simulink model "hexacopter_sim"  (R2023a)
settings: Solver=VariableStepAuto  StartTime=0.0  StopTime=15  MaxStep=0.001  RelTol=1e-7  EnableMultiTasking=on
values from neighbouring files (symbols this model uses):
  arm_length = 0.35    [hexacopter.m]    (also in hexacopter_unmodified.m)
  batteryDistanceFromCOG = -0.1    [hexacopter.m]    (also in hexacopter_unmodified.m)
  batteryMass = 0.56*2    (= 1.12)    [hexacopter.m]    (also in hexacopter_unmodified.m)
  batVolt = 3.7*cells    (= 14.8)    [hexacopter.m]    (also in hexacopter_unmodified.m)
  bodyMass = 1.2    [hexacopter.m]    (also in hexacopter_unmodified.m)
  deadCurrent = 0.3    [hexacopter.m]    (also in hexacopter_unmodified.m)
  droneMass = bodyMass + motorCount*(motorMass + propellerMassRaw)    (= 2.424)    [hexacopter.m]    (also in hexacopter_unmodified.m)
  h1al = 0.07    [discrete_controller_tuning.m]    (also in height_controller.m; hexacopter.m; hexacopter_unmodified.m)
  h1kp = 60    [hexacopter.m]    (also in hexacopter_unmodified.m)
  h1td = 1 / (sqrt(h1al) * target)    [height_controller.m]    (also in hexacopter.m = 1; hexacopter_unmodified.m = 1)
  h1ti = h1Ni * (1/ target)    (= 1.27118644068)    [height_controller.m]    (also in hexacopter.m = 1; hexacopter_unmodified.m = 1)
  h1val = 0.6    [discrete_controller_tuning.m]    (also in hexacopter.m = 0)
  h1vkp = 1    [hexacopter.m]
  h1vtd = 0    [hexacopter.m]
  h1vti = 1    [hexacopter.m]
  h_beta = 5    [hexacopter.m]    (also in hexacopter_unmodified.m)
  h_tau = 1.5    [hexacopter.m]    (also in hexacopter_unmodified.m)
  hoverControl = hoverVoltage/batVolt*1024    [hexacopter.m]    (also in hexacopter_unmodified.m)
  hoverVoltage = hoverCurrent * Ra + hoverRPM / Kv    [hexacopter.m]    (also in hexacopter_unmodified.m)
  KDrag = 1.5e-9    (= 1.5e-09)    [hexacopter.m]    (also in hexacopter_unmodified.m)
  Km = 60/(Kv * 2 * pi)    (= 0.013641852265)    [hexacopter.m]    (also in hexacopter_unmodified.m)
  Ktrust = 2.7e-5    (= 2.7e-05)    [hexacopter.m]    (also in hexacopter_unmodified.m)
  minimumMotorVolt = 1.0    (= 1)    [hexacopter.m]    (also in hexacopter_unmodified.m)
  motorMass = motorOnlyMass + 0.085    (= 0.187)    [hexacopter.m]    (also in hexacopter_unmodified.m)
  N = solve(eqn,V)    [temp.m]
  paal = 0.2    [hexacopter.m]    (also in hexacopter_unmodified.m)
  pakp = 0    [hexacopter.m]    (also in hexacopter_unmodified.m)
  pal = 0.5    [hexacopter.m]    (also in hexacopter_unmodified.m)
  patd = 1    [hexacopter.m]    (also in hexacopter_unmodified.m)
  pati = 100    [hexacopter.m]    (also in hexacopter_unmodified.m)
  pkp = 0    [hexacopter.m]    (also in hexacopter_unmodified.m)
  propellerMass = propellerMassRaw + 3*motorInertia/propellerRadius^2    (= 0.0220980494455)    [hexacopter.m]    (also in hexacopter_unmodified.m)
  ptd = 1    [hexacopter.m]    (also in hexacopter_unmodified.m)
  pti = 1    [hexacopter.m]    (also in hexacopter_unmodified.m)
  pushEnabled = 0    [hexacopter.m]    (also in hexacopter_unmodified.m)
  Ra = 0.083    [hexacopter.m]    (also in hexacopter_unmodified.m)
  raal = 0.2    [hexacopter.m]    (also in hexacopter_unmodified.m)
  rakp = 0    [hexacopter.m]    (also in hexacopter_unmodified.m)
  ral = 0.5    [hexacopter.m]    (also in hexacopter_unmodified.m)
  ratd = 1    [hexacopter.m]    (also in hexacopter_unmodified.m)
  rati = 100    [hexacopter.m]    (also in hexacopter_unmodified.m)
  rkp = 0    [hexacopter.m]    (also in hexacopter_unmodified.m)
  roll_limit = 10    [hexacopter.m]    (also in hexacopter_unmodified.m)
  rtd = 1    [hexacopter.m]    (also in hexacopter_unmodified.m)
  rti = 1    [hexacopter.m]    (also in hexacopter_unmodified.m)
  xal = 0.2    [hexacopter.m]    (also in hexacopter_unmodified.m = 1)
  xkp = 0    [hexacopter.m]    (also in hexacopter_unmodified.m)
  xtd = 1    [hexacopter.m]    (also in hexacopter_unmodified.m)
  xti = 100    [hexacopter.m]    (also in hexacopter_unmodified.m)
  xval = 0.2    [hexacopter.m]    (also in hexacopter_unmodified.m = 0.3; vel_controller.m = 0.3)
  xvkp = 0    [hexacopter.m]    (also in hexacopter_unmodified.m; vel_controller.m = 0.184077200147)
  xvtd = 1    [hexacopter.m]    (also in hexacopter_unmodified.m; vel_controller.m = 1 / (sqrt(xval) * target))
  xvti = 100    [hexacopter.m]    (also in hexacopter_unmodified.m; vel_controller.m = 0)
  yaal = 0.5    [hexacopter.m]    (also in hexacopter_unmodified.m)
  yakp = 0    [hexacopter.m]    (also in hexacopter_unmodified.m)
  yal = 0.5    [hexacopter.m]    (also in hexacopter_unmodified.m)
  yatd = 1    [hexacopter.m]    (also in hexacopter_unmodified.m)
  yati = 100    [hexacopter.m]    (also in hexacopter_unmodified.m)
  yaw_limit = 45    [hexacopter.m]    (also in hexacopter_unmodified.m)
  yiLim = 500    [hexacopter.m]    (also in hexacopter_unmodified.m)
  ykp = 0    [hexacopter.m]    (also in hexacopter_unmodified.m)
  ytd = 0    [hexacopter.m]    (also in hexacopter_unmodified.m)
  yti = 1000    [hexacopter.m]    (also in hexacopter_unmodified.m)
  yval = 0.3    [hexacopter.m]    (also in hexacopter_unmodified.m)
  yvkp = 0    [hexacopter.m]    (also in hexacopter_unmodified.m)
  yvtd = 1    [hexacopter.m]    (also in hexacopter_unmodified.m)
  yvti = 100    [hexacopter.m]    (also in hexacopter_unmodified.m)
undefined symbols (not defined in the file or in its folder): h2al, h2kp, h2td, h2ti, X, Y, Z
libraries: sm_lib x52, nesl_utility x34, simulink x3
(part 3 of 3)

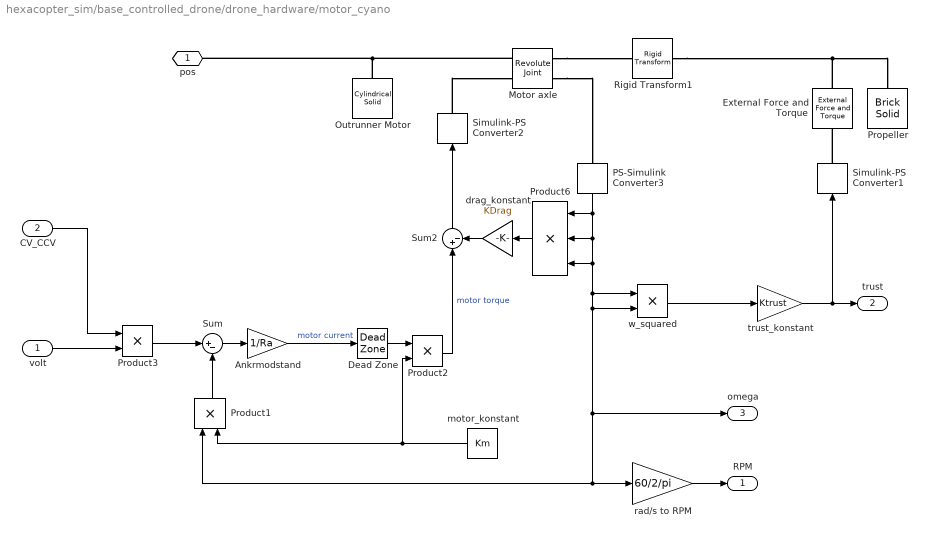
== system hexacopter_sim/base_controlled_drone/drone_hardware/motor_cyano ==
  volt : Inport
  CV_CCV : Inport  Port=2
  Ankrmodstand : Gain  Gain=1/Ra
  Dead Zone : DeadZone  LowerValue=-deadCurrent  UpperValue=deadCurrent
  External Force and Torque : sm_lib/Forces and Torques/External Force and Torque  ForceResolutionFrame=AttachedFrame  EnableForceX=off  EnableForceY=off  EnableForceZ=on  EnableForce=off  TorqueResolutionFrame=AttachedFrame  EnableTorqueX=off  EnableTorqueY=off  EnableTorqueZ=off  EnableTorque=off
  Motor axle : sm_lib/Joints/Revolute Joint  JointMode=Normal  SenseConstraintForce=off  SenseConstraintForceX=off  SenseConstraintForceY=off  SenseConstraintForceZ=off  SenseConstraintTorque=off  SenseConstraintTorqueX=off  SenseConstraintTorqueY=off  SenseConstraintTorqueZ=off  SenseTotalForce=off  SenseTotalForceX=off  SenseTotalForceY=off  SenseTotalForceZ=off  SenseTotalTorque=off  SenseTotalTorqueX=off  SenseTotalTorqueY=off  SenseTotalTorqueZ=off  CompositeWrenchDir=FollowerOnBase  CompositeWrenchFrame=BaseFrame  EquilibriumPosition=0  EquilibriumPositionUnits=deg  SpringStiffness=0  SpringStiffnessUnits=N*m/deg  DampingCoefficient=0  DampingCoefficientUnits=N*m/(deg/s)  TorqueActuationMode=InputTorque  MotionActuationMode=ComputedMotion  SensePosition=off  SenseVelocity=on  SenseAcceleration=off  SenseTorqueForce=off  SenseLowerLimitTorqueForce=off  SenseUpperLimitTorqueForce=off  LowerLimitSpecify=off  LowerLimitBound=-90  LowerLimitBoundUnits=deg  LowerLimitStiffness=1e4  LowerLimitStiffnessUnits=N*m/deg  LowerLimitDamping=10  LowerLimitDampingUnits=N*m/(deg/s)  LowerLimitTransitionRegionWidth=0.1  LowerLimitTransitionRegionWidthUnits=deg  UpperLimitSpecify=off  UpperLimitBound=90  UpperLimitBoundUnits=deg  UpperLimitStiffness=1e4  UpperLimitStiffnessUnits=N*m/deg  UpperLimitDamping=10  UpperLimitDampingUnits=N*m/(deg/s)  UpperLimitTransitionRegionWidth=0.1  UpperLimitTransitionRegionWidthUnits=deg  PositionTargetSpecify=off  PositionTargetPriority=High  PositionTargetValue=0  PositionTargetValueUnits=deg  VelocityTargetSpecify=on  VelocityTargetPriority=High  VelocityTargetValue=0  VelocityTargetValueUnits=rad/s
  Outrunner Motor : sm_lib/Body Elements/Cylindrical Solid  GraphicAmbientColor=[0.15 0.15 0.15 1.0]  BasedOnType=Mass  CenterOfMass=[0 0 0]  CenterOfMassUnits=m  GraphicDiffuseColor=[0.2 0.6 0.0]  CylinderLength=0.05  CylinderLengthUnits=m  CylinderRadius=0.02  CylinderRadiusUnits=m  Density=1000  DensityUnits=kg/(m^3)  DoExposeReferenceFrame=on  GraphicEmissiveColor=[0.0 0.0 0.0 1.0]  ExportEntireGeometry=off  SerializedFrames=<Frames/>  MarkerShape=Sphere  MarkerSize=10  GraphicType=FromGeometry  InertiaType=CalculateFromGeometry  Mass=motorMass  MassUnits=kg  MomentsOfInertia=[1 1 1]  MomentsOfInertiaUnits=kg*m^2  GraphicOpacity=1.0  ProductsOfInertia=[0 0 0]  ProductsOfInertiaUnits=kg*m^2  GraphicShininess=75  GraphicSpecularColor=[0.5 0.5 0.5 1.0]  GraphicVisPropType=SimpleVisualProperties
  PS-Simulink Converter3 : nesl_utility/PS-Simulink Converter  PhysicalDomain=network_engine_domain  SubClassName=ps_output  LeftPortType=input  RightPortType=output  PseudoPeriodic=off  Frequencies=[]  VectorFormat=1-D array  Unit=1  AffineConversion=off
  Product1 : Product
  Product2 : Product
  Product3 : Product
  Product6 : Product  Inputs=3
  Propeller : sm_lib/Body Elements/Brick Solid  GraphicAmbientColor=[0.15 0.15 0.15 1.0]  BasedOnType=Mass  BrickDimensions=[0.34 0.03 0.01]  BrickDimensionsUnits=m  CenterOfMass=[0 0 0]  CenterOfMassUnits=m  GraphicDiffuseColor=[0.0 0.8 0.8]  Density=1000  DensityUnits=kg/(m^3)  DoExposeReferenceFrame=on  GraphicEmissiveColor=[0.0 0.0 0.0 1.0]  ExportEntireGeometry=off  SerializedFrames=<Frames/>  MarkerShape=Sphere  MarkerSize=10  GraphicType=FromGeometry  InertiaType=CalculateFromGeometry  Mass=propellerMass  MassUnits=kg  MomentsOfInertia=[1 1 1]  MomentsOfInertiaUnits=kg*m^2  GraphicOpacity=1.0  ProductsOfInertia=[0 0 0]  ProductsOfInertiaUnits=kg*m^2  GraphicShininess=75  GraphicSpecularColor=[0.5 0.5 0.5 1.0]  GraphicVisPropType=SimpleVisualProperties
  Rigid Transform1 : sm_lib/Frames and Transforms/Rigid Transform  TranslationMethod=Cartesian  TranslationStandardOffset=0  TranslationStandardOffsetUnits=m  TranslationStandardAxis=+Z  TranslationCartesianOffset=[0 0 0.03]  TranslationCartesianOffsetUnits=m  TranslationROffset=0  TranslationROffsetUnits=m  TranslationZOffset=0  TranslationZOffsetUnits=m  TranslationThetaOffset=0  TranslationThetaOffsetUnits=deg  RotationMethod=StandardAxis  RotationAngleUnits=deg  RotationStandardAxis=+Z  RotationAngle=0.0  RotationArbitraryAxis=[0 0 1]  FollAlignAxisA=+X  BaseAlignAxisA=+Y  FollAlignAxisB=+Y  BaseAlignAxisB=+Z  RotationSequenceAxes=FollowerAxes  RotationSequence=XYX  RotationSequenceAngles=[0 0 0]  RotationSequenceAnglesUnits=deg  RotationMatrix=[1 0 0; 0 1 0; 0 0 1]  Quaternion=[1 0 0 0]
  Simulink-PS Converter1 : nesl_utility/Simulink-PS Converter  PhysicalDomain=network_engine_domain  SubClassName=ps_input  LeftPortType=input  RightPortType=output  PseudoPeriodic=off  Frequencies=[]  NoiseDistribution=none  NoiseParameters=[]  Unit=1  AffineConversion=off  FilteringAndDerivatives=zero  SimscapeFilterOrder=1  InputFilterTimeConstant=0.001  UdotUserProvided=1
  Simulink-PS Converter2 : nesl_utility/Simulink-PS Converter  PhysicalDomain=network_engine_domain  SubClassName=ps_input  LeftPortType=input  RightPortType=output  PseudoPeriodic=off  Frequencies=[]  NoiseDistribution=none  NoiseParameters=[]  Unit=1  AffineConversion=off  FilteringAndDerivatives=zero  SimscapeFilterOrder=1  InputFilterTimeConstant=0.001  UdotUserProvided=1
  Sum : Sum  Inputs=|+-
  Sum2 : Sum  Inputs=|+-
  drag_konstant : Gain  Gain=KDrag
  motor_konstant : Constant  Value=Km
  rad/s to RPM : Gain  Gain=60/2/pi
  trust_konstant : Gain  Gain=Ktrust
  w_squared : Product
  pos : PMIOPort  Side=Left
  RPM : Outport  VectorParamsAs1DForOutWhenUnconnected=off
  trust : Outport  Port=2  VectorParamsAs1DForOutWhenUnconnected=off
  omega : Outport  Port=3  VectorParamsAs1DForOutWhenUnconnected=off
  wires:
  rad/s to RPM/1 -> RPM/1
  motor_konstant/1 -> Product1/2, Product2/2
  Product1/1 -> Sum/2
  Product2/1 -> Sum2/1  "motor torque"
  Ankrmodstand/1 -> Dead Zone/1  "motor current"
  Sum/1 -> Ankrmodstand/1
  Sum2/1 -> Simulink-PS Converter2/1
  drag_konstant/1 -> Sum2/2
  volt/1 -> Product3/2
  Product3/1 -> Sum/1
  CV_CCV/1 -> Product3/1
  trust_konstant/1 -> trust/1, Simulink-PS Converter1/1
  w_squared/1 -> trust_konstant/1
  PS-Simulink Converter3/1 -> Product6/2, Product6/3, omega/1, rad/s to RPM/1, Product1/1, w_squared/2, w_squared/1, Product6/1
  Product6/1 -> drag_konstant/1
  Dead Zone/1 -> Product2/1
  connections:
  Simulink-PS Converter1/RConn1 -- External Force and Torque/LConn1
  Motor axle/RConn2 -- PS-Simulink Converter3/LConn1
  Motor axle/RConn1 -- Rigid Transform1/LConn1
  Simulink-PS Converter2/RConn1 -- Motor axle/LConn2
  Motor axle/LConn1 -- Outrunner Motor/RConn1 -- pos/RConn1
  External Force and Torque/RConn1 -- Propeller/RConn1 -- Rigid Transform1/RConn1

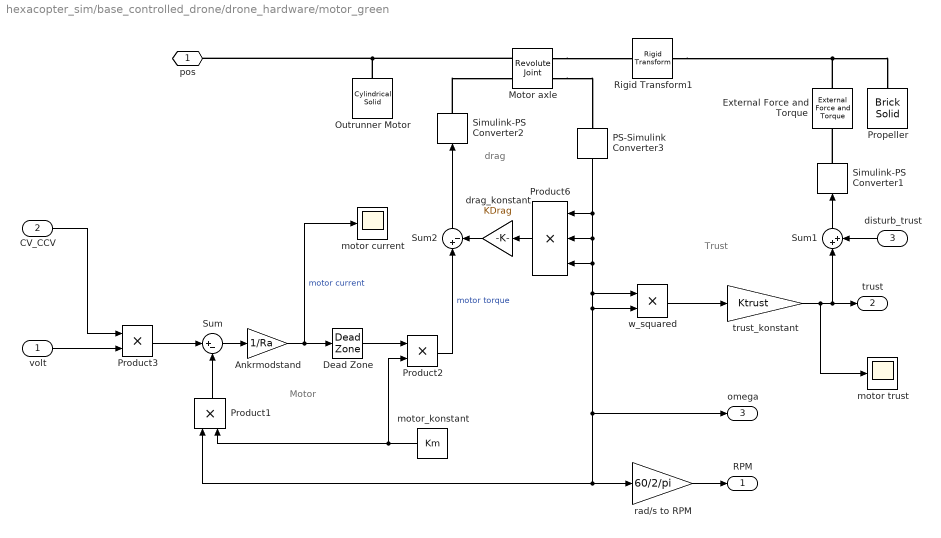
== system hexacopter_sim/base_controlled_drone/drone_hardware/motor_green ==
  note: drag
  note: Trust
  note: Motor
  volt : Inport
  CV_CCV : Inport  Port=2
  disturb_trust : Inport  Port=3
  Ankrmodstand : Gain  Gain=1/Ra
  Dead Zone : DeadZone  LowerValue=-deadCurrent  UpperValue=deadCurrent
  External Force and Torque : sm_lib/Forces and Torques/External Force and Torque  ForceResolutionFrame=AttachedFrame  EnableForceX=off  EnableForceY=off  EnableForceZ=on  EnableForce=off  TorqueResolutionFrame=AttachedFrame  EnableTorqueX=off  EnableTorqueY=off  EnableTorqueZ=off  EnableTorque=off
  Motor axle : sm_lib/Joints/Revolute Joint  JointMode=Normal  SenseConstraintForce=off  SenseConstraintForceX=off  SenseConstraintForceY=off  SenseConstraintForceZ=off  SenseConstraintTorque=off  SenseConstraintTorqueX=off  SenseConstraintTorqueY=off  SenseConstraintTorqueZ=off  SenseTotalForce=off  SenseTotalForceX=off  SenseTotalForceY=off  SenseTotalForceZ=off  SenseTotalTorque=off  SenseTotalTorqueX=off  SenseTotalTorqueY=off  SenseTotalTorqueZ=off  CompositeWrenchDir=FollowerOnBase  CompositeWrenchFrame=BaseFrame  EquilibriumPosition=0  EquilibriumPositionUnits=deg  SpringStiffness=0  SpringStiffnessUnits=N*m/deg  DampingCoefficient=0  DampingCoefficientUnits=N*m/(deg/s)  TorqueActuationMode=InputTorque  MotionActuationMode=ComputedMotion  SensePosition=off  SenseVelocity=on  SenseAcceleration=off  SenseTorqueForce=off  SenseLowerLimitTorqueForce=off  SenseUpperLimitTorqueForce=off  LowerLimitSpecify=off  LowerLimitBound=-90  LowerLimitBoundUnits=deg  LowerLimitStiffness=1e4  LowerLimitStiffnessUnits=N*m/deg  LowerLimitDamping=10  LowerLimitDampingUnits=N*m/(deg/s)  LowerLimitTransitionRegionWidth=0.1  LowerLimitTransitionRegionWidthUnits=deg  UpperLimitSpecify=off  UpperLimitBound=90  UpperLimitBoundUnits=deg  UpperLimitStiffness=1e4  UpperLimitStiffnessUnits=N*m/deg  UpperLimitDamping=10  UpperLimitDampingUnits=N*m/(deg/s)  UpperLimitTransitionRegionWidth=0.1  UpperLimitTransitionRegionWidthUnits=deg  PositionTargetSpecify=off  PositionTargetPriority=High  PositionTargetValue=0  PositionTargetValueUnits=deg  VelocityTargetSpecify=on  VelocityTargetPriority=High  VelocityTargetValue=0  VelocityTargetValueUnits=rad/s
  Outrunner Motor : sm_lib/Body Elements/Cylindrical Solid  GraphicAmbientColor=[0.15 0.15 0.15 1.0]  BasedOnType=Mass  CenterOfMass=[0 0 0]  CenterOfMassUnits=m  GraphicDiffuseColor=[0.2 0.6 0.0]  CylinderLength=0.05  CylinderLengthUnits=m  CylinderRadius=0.02  CylinderRadiusUnits=m  Density=1000  DensityUnits=kg/(m^3)  DoExposeReferenceFrame=on  GraphicEmissiveColor=[0.0 0.0 0.0 1.0]  ExportEntireGeometry=off  SerializedFrames=<Frames/>  MarkerShape=Sphere  MarkerSize=10  GraphicType=FromGeometry  InertiaType=CalculateFromGeometry  Mass=motorMass  MassUnits=kg  MomentsOfInertia=[1 1 1]  MomentsOfInertiaUnits=kg*m^2  GraphicOpacity=1.0  ProductsOfInertia=[0 0 0]  ProductsOfInertiaUnits=kg*m^2  GraphicShininess=75  GraphicSpecularColor=[0.5 0.5 0.5 1.0]  GraphicVisPropType=SimpleVisualProperties
  PS-Simulink Converter3 : nesl_utility/PS-Simulink Converter  PhysicalDomain=network_engine_domain  SubClassName=ps_output  LeftPortType=input  RightPortType=output  PseudoPeriodic=off  Frequencies=[]  VectorFormat=1-D array  Unit=1  AffineConversion=off
  Product1 : Product
  Product2 : Product
  Product3 : Product
  Product6 : Product  Inputs=3
  Propeller : sm_lib/Body Elements/Brick Solid  GraphicAmbientColor=[0.15 0.15 0.15 1.0]  BasedOnType=Mass  BrickDimensions=[0.34 0.03 0.01]  BrickDimensionsUnits=m  CenterOfMass=[0 0 0]  CenterOfMassUnits=m  GraphicDiffuseColor=[0.0 0.8 0.0]  Density=1000  DensityUnits=kg/(m^3)  DoExposeReferenceFrame=on  GraphicEmissiveColor=[0.0 0.0 0.0 1.0]  ExportEntireGeometry=off  SerializedFrames=<Frames/>  MarkerShape=Sphere  MarkerSize=10  GraphicType=FromGeometry  InertiaType=CalculateFromGeometry  Mass=propellerMass  MassUnits=kg  MomentsOfInertia=[1 1 1]  MomentsOfInertiaUnits=kg*m^2  GraphicOpacity=1.0  ProductsOfInertia=[0 0 0]  ProductsOfInertiaUnits=kg*m^2  GraphicShininess=75  GraphicSpecularColor=[0.5 0.5 0.5 1.0]  GraphicVisPropType=SimpleVisualProperties
  Rigid Transform1 : sm_lib/Frames and Transforms/Rigid Transform  TranslationMethod=Cartesian  TranslationStandardOffset=0  TranslationStandardOffsetUnits=m  TranslationStandardAxis=+Z  TranslationCartesianOffset=[0 0 0.03]  TranslationCartesianOffsetUnits=m  TranslationROffset=0  TranslationROffsetUnits=m  TranslationZOffset=0  TranslationZOffsetUnits=m  TranslationThetaOffset=0  TranslationThetaOffsetUnits=deg  RotationMethod=StandardAxis  RotationAngleUnits=deg  RotationStandardAxis=+Z  RotationAngle=0.0  RotationArbitraryAxis=[0 0 1]  FollAlignAxisA=+X  BaseAlignAxisA=+Y  FollAlignAxisB=+Y  BaseAlignAxisB=+Z  RotationSequenceAxes=FollowerAxes  RotationSequence=XYX  RotationSequenceAngles=[0 0 0]  RotationSequenceAnglesUnits=deg  RotationMatrix=[1 0 0; 0 1 0; 0 0 1]  Quaternion=[1 0 0 0]
  Simulink-PS Converter1 : nesl_utility/Simulink-PS Converter  PhysicalDomain=network_engine_domain  SubClassName=ps_input  LeftPortType=input  RightPortType=output  PseudoPeriodic=off  Frequencies=[]  NoiseDistribution=none  NoiseParameters=[]  Unit=1  AffineConversion=off  FilteringAndDerivatives=zero  SimscapeFilterOrder=1  InputFilterTimeConstant=0.001  UdotUserProvided=1
  Simulink-PS Converter2 : nesl_utility/Simulink-PS Converter  PhysicalDomain=network_engine_domain  SubClassName=ps_input  LeftPortType=input  RightPortType=output  PseudoPeriodic=off  Frequencies=[]  NoiseDistribution=none  NoiseParameters=[]  Unit=1  AffineConversion=off  FilteringAndDerivatives=zero  SimscapeFilterOrder=1  InputFilterTimeConstant=0.001  UdotUserProvided=1
  Sum : Sum  Inputs=|+-
  Sum1 : Sum  Inputs=|++
  Sum2 : Sum  Inputs=|+-
  drag_konstant : Gain  Gain=KDrag
  motor current : Scope
  motor trust : Scope
  motor_konstant : Constant  Value=Km
  rad/s to RPM : Gain  Gain=60/2/pi
  trust_konstant : Gain  Gain=Ktrust
  w_squared : Product
  pos : PMIOPort  Side=Left
  RPM : Outport  VectorParamsAs1DForOutWhenUnconnected=off
  trust : Outport  Port=2  VectorParamsAs1DForOutWhenUnconnected=off
  omega : Outport  Port=3  VectorParamsAs1DForOutWhenUnconnected=off
  wires:
  rad/s to RPM/1 -> RPM/1
  motor_konstant/1 -> Product1/2, Product2/2
  Product1/1 -> Sum/2
  trust_konstant/1 -> motor trust/1, Sum1/1, trust/1
  Product2/1 -> Sum2/1  "motor torque"
  Ankrmodstand/1 -> motor current/1, Dead Zone/1  "motor current"
  Sum/1 -> Ankrmodstand/1
  Sum2/1 -> Simulink-PS Converter2/1
  drag_konstant/1 -> Sum2/2
  volt/1 -> Product3/2
  Product3/1 -> Sum/1
  CV_CCV/1 -> Product3/1
  Sum1/1 -> Simulink-PS Converter1/1
  disturb_trust/1 -> Sum1/2
  w_squared/1 -> trust_konstant/1
  PS-Simulink Converter3/1 -> omega/1, rad/s to RPM/1, Product1/1, w_squared/2, w_squared/1, Product6/3, Product6/2, Product6/1
  Product6/1 -> drag_konstant/1
  Dead Zone/1 -> Product2/1
  connections:
  Simulink-PS Converter1/RConn1 -- External Force and Torque/LConn1
  Motor axle/RConn2 -- PS-Simulink Converter3/LConn1
  Motor axle/RConn1 -- Rigid Transform1/LConn1
  Simulink-PS Converter2/RConn1 -- Motor axle/LConn2
  Motor axle/LConn1 -- Outrunner Motor/RConn1 -- pos/RConn1
  External Force and Torque/RConn1 -- Propeller/RConn1 -- Rigid Transform1/RConn1

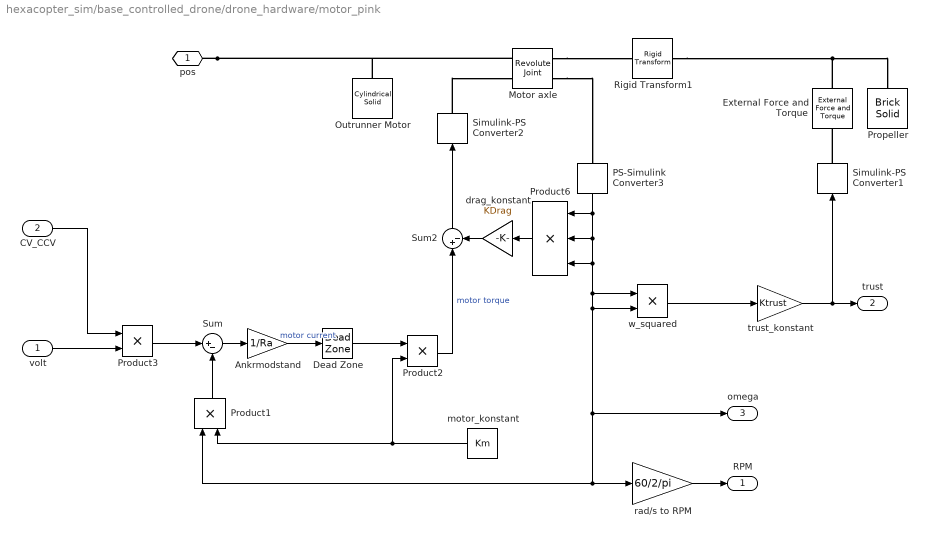
== system hexacopter_sim/base_controlled_drone/drone_hardware/motor_pink ==
  volt : Inport
  CV_CCV : Inport  Port=2
  Ankrmodstand : Gain  Gain=1/Ra
  Dead Zone : DeadZone  LowerValue=-deadCurrent  UpperValue=deadCurrent
  External Force and Torque : sm_lib/Forces and Torques/External Force and Torque  ForceResolutionFrame=AttachedFrame  EnableForceX=off  EnableForceY=off  EnableForceZ=on  EnableForce=off  TorqueResolutionFrame=AttachedFrame  EnableTorqueX=off  EnableTorqueY=off  EnableTorqueZ=off  EnableTorque=off
  Motor axle : sm_lib/Joints/Revolute Joint  JointMode=Normal  SenseConstraintForce=off  SenseConstraintForceX=off  SenseConstraintForceY=off  SenseConstraintForceZ=off  SenseConstraintTorque=off  SenseConstraintTorqueX=off  SenseConstraintTorqueY=off  SenseConstraintTorqueZ=off  SenseTotalForce=off  SenseTotalForceX=off  SenseTotalForceY=off  SenseTotalForceZ=off  SenseTotalTorque=off  SenseTotalTorqueX=off  SenseTotalTorqueY=off  SenseTotalTorqueZ=off  CompositeWrenchDir=FollowerOnBase  CompositeWrenchFrame=BaseFrame  EquilibriumPosition=0  EquilibriumPositionUnits=deg  SpringStiffness=0  SpringStiffnessUnits=N*m/deg  DampingCoefficient=0  DampingCoefficientUnits=N*m/(deg/s)  TorqueActuationMode=InputTorque  MotionActuationMode=ComputedMotion  SensePosition=off  SenseVelocity=on  SenseAcceleration=off  SenseTorqueForce=off  SenseLowerLimitTorqueForce=off  SenseUpperLimitTorqueForce=off  LowerLimitSpecify=off  LowerLimitBound=-90  LowerLimitBoundUnits=deg  LowerLimitStiffness=1e4  LowerLimitStiffnessUnits=N*m/deg  LowerLimitDamping=10  LowerLimitDampingUnits=N*m/(deg/s)  LowerLimitTransitionRegionWidth=0.1  LowerLimitTransitionRegionWidthUnits=deg  UpperLimitSpecify=off  UpperLimitBound=90  UpperLimitBoundUnits=deg  UpperLimitStiffness=1e4  UpperLimitStiffnessUnits=N*m/deg  UpperLimitDamping=10  UpperLimitDampingUnits=N*m/(deg/s)  UpperLimitTransitionRegionWidth=0.1  UpperLimitTransitionRegionWidthUnits=deg  PositionTargetSpecify=off  PositionTargetPriority=High  PositionTargetValue=0  PositionTargetValueUnits=deg  VelocityTargetSpecify=on  VelocityTargetPriority=High  VelocityTargetValue=0  VelocityTargetValueUnits=rad/s
  Outrunner Motor : sm_lib/Body Elements/Cylindrical Solid  GraphicAmbientColor=[0.15 0.15 0.15 1.0]  BasedOnType=Mass  CenterOfMass=[0 0 0]  CenterOfMassUnits=m  GraphicDiffuseColor=[0.2 0.6 0.0]  CylinderLength=0.05  CylinderLengthUnits=m  CylinderRadius=0.02  CylinderRadiusUnits=m  Density=1000  DensityUnits=kg/(m^3)  DoExposeReferenceFrame=on  GraphicEmissiveColor=[0.0 0.0 0.0 1.0]  ExportEntireGeometry=off  SerializedFrames=<Frames/>  MarkerShape=Sphere  MarkerSize=10  GraphicType=FromGeometry  InertiaType=CalculateFromGeometry  Mass=motorMass  MassUnits=kg  MomentsOfInertia=[1 1 1]  MomentsOfInertiaUnits=kg*m^2  GraphicOpacity=1.0  ProductsOfInertia=[0 0 0]  ProductsOfInertiaUnits=kg*m^2  GraphicShininess=75  GraphicSpecularColor=[0.5 0.5 0.5 1.0]  GraphicVisPropType=SimpleVisualProperties
  PS-Simulink Converter3 : nesl_utility/PS-Simulink Converter  PhysicalDomain=network_engine_domain  SubClassName=ps_output  LeftPortType=input  RightPortType=output  PseudoPeriodic=off  Frequencies=[]  VectorFormat=1-D array  Unit=1  AffineConversion=off
  Product1 : Product
  Product2 : Product
  Product3 : Product
  Product6 : Product  Inputs=3
  Propeller : sm_lib/Body Elements/Brick Solid  GraphicAmbientColor=[0.15 0.15 0.15 1.0]  BasedOnType=Mass  BrickDimensions=[0.34 0.03 0.01]  BrickDimensionsUnits=m  CenterOfMass=[0 0 0]  CenterOfMassUnits=m  GraphicDiffuseColor=[0.9 0.6 0.6]  Density=1000  DensityUnits=kg/(m^3)  DoExposeReferenceFrame=on  GraphicEmissiveColor=[0.0 0.0 0.0 1.0]  ExportEntireGeometry=off  SerializedFrames=<Frames/>  MarkerShape=Sphere  MarkerSize=10  GraphicType=FromGeometry  InertiaType=CalculateFromGeometry  Mass=propellerMass  MassUnits=kg  MomentsOfInertia=[1 1 1]  MomentsOfInertiaUnits=kg*m^2  GraphicOpacity=1.0  ProductsOfInertia=[0 0 0]  ProductsOfInertiaUnits=kg*m^2  GraphicShininess=75  GraphicSpecularColor=[0.5 0.5 0.5 1.0]  GraphicVisPropType=SimpleVisualProperties
  Rigid Transform1 : sm_lib/Frames and Transforms/Rigid Transform  TranslationMethod=Cartesian  TranslationStandardOffset=0  TranslationStandardOffsetUnits=m  TranslationStandardAxis=+Z  TranslationCartesianOffset=[0 0 0.03]  TranslationCartesianOffsetUnits=m  TranslationROffset=0  TranslationROffsetUnits=m  TranslationZOffset=0  TranslationZOffsetUnits=m  TranslationThetaOffset=0  TranslationThetaOffsetUnits=deg  RotationMethod=StandardAxis  RotationAngleUnits=deg  RotationStandardAxis=+Z  RotationAngle=0.0  RotationArbitraryAxis=[0 0 1]  FollAlignAxisA=+X  BaseAlignAxisA=+Y  FollAlignAxisB=+Y  BaseAlignAxisB=+Z  RotationSequenceAxes=FollowerAxes  RotationSequence=XYX  RotationSequenceAngles=[0 0 0]  RotationSequenceAnglesUnits=deg  RotationMatrix=[1 0 0; 0 1 0; 0 0 1]  Quaternion=[1 0 0 0]
  Simulink-PS Converter1 : nesl_utility/Simulink-PS Converter  PhysicalDomain=network_engine_domain  SubClassName=ps_input  LeftPortType=input  RightPortType=output  PseudoPeriodic=off  Frequencies=[]  NoiseDistribution=none  NoiseParameters=[]  Unit=1  AffineConversion=off  FilteringAndDerivatives=zero  SimscapeFilterOrder=1  InputFilterTimeConstant=0.001  UdotUserProvided=1
  Simulink-PS Converter2 : nesl_utility/Simulink-PS Converter  PhysicalDomain=network_engine_domain  SubClassName=ps_input  LeftPortType=input  RightPortType=output  PseudoPeriodic=off  Frequencies=[]  NoiseDistribution=none  NoiseParameters=[]  Unit=1  AffineConversion=off  FilteringAndDerivatives=zero  SimscapeFilterOrder=1  InputFilterTimeConstant=0.001  UdotUserProvided=1
  Sum : Sum  Inputs=|+-
  Sum2 : Sum  Inputs=|+-
  drag_konstant : Gain  Gain=KDrag
  motor_konstant : Constant  Value=Km
  rad/s to RPM : Gain  Gain=60/2/pi
  trust_konstant : Gain  Gain=Ktrust
  w_squared : Product
  pos : PMIOPort  Side=Left
  RPM : Outport  VectorParamsAs1DForOutWhenUnconnected=off
  trust : Outport  Port=2  VectorParamsAs1DForOutWhenUnconnected=off
  omega : Outport  Port=3  VectorParamsAs1DForOutWhenUnconnected=off
  wires:
  Product6/1 -> drag_konstant/1
  PS-Simulink Converter3/1 -> Product6/1, Product6/2, Product6/3, w_squared/1, w_squared/2, Product1/1, rad/s to RPM/1, omega/1
  w_squared/1 -> trust_konstant/1
  trust_konstant/1 -> Simulink-PS Converter1/1, trust/1
  CV_CCV/1 -> Product3/1
  Product3/1 -> Sum/1
  volt/1 -> Product3/2
  drag_konstant/1 -> Sum2/2
  Sum2/1 -> Simulink-PS Converter2/1
  Sum/1 -> Ankrmodstand/1
  Ankrmodstand/1 -> Dead Zone/1  "motor current"
  Product2/1 -> Sum2/1  "motor torque"
  Product1/1 -> Sum/2
  motor_konstant/1 -> Product1/2, Product2/2
  rad/s to RPM/1 -> RPM/1
  Dead Zone/1 -> Product2/1
  connections:
  Rigid Transform1/RConn1 -- Propeller/RConn1 -- External Force and Torque/RConn1
  pos/RConn1 -- Outrunner Motor/RConn1 -- Motor axle/LConn1
  Simulink-PS Converter2/RConn1 -- Motor axle/LConn2
  Motor axle/RConn1 -- Rigid Transform1/LConn1
  Motor axle/RConn2 -- PS-Simulink Converter3/LConn1
  Simulink-PS Converter1/RConn1 -- External Force and Torque/LConn1

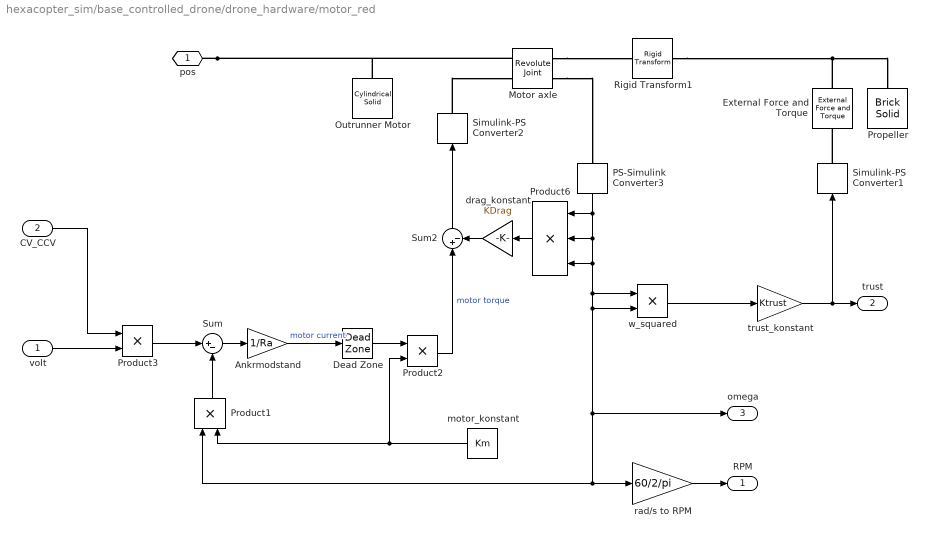
== system hexacopter_sim/base_controlled_drone/drone_hardware/motor_red ==
  volt : Inport
  CV_CCV : Inport  Port=2
  Ankrmodstand : Gain  Gain=1/Ra
  Dead Zone : DeadZone  LowerValue=-deadCurrent  UpperValue=deadCurrent
  External Force and Torque : sm_lib/Forces and Torques/External Force and Torque  ForceResolutionFrame=AttachedFrame  EnableForceX=off  EnableForceY=off  EnableForceZ=on  EnableForce=off  TorqueResolutionFrame=AttachedFrame  EnableTorqueX=off  EnableTorqueY=off  EnableTorqueZ=off  EnableTorque=off
  Motor axle : sm_lib/Joints/Revolute Joint  JointMode=Normal  SenseConstraintForce=off  SenseConstraintForceX=off  SenseConstraintForceY=off  SenseConstraintForceZ=off  SenseConstraintTorque=off  SenseConstraintTorqueX=off  SenseConstraintTorqueY=off  SenseConstraintTorqueZ=off  SenseTotalForce=off  SenseTotalForceX=off  SenseTotalForceY=off  SenseTotalForceZ=off  SenseTotalTorque=off  SenseTotalTorqueX=off  SenseTotalTorqueY=off  SenseTotalTorqueZ=off  CompositeWrenchDir=FollowerOnBase  CompositeWrenchFrame=BaseFrame  EquilibriumPosition=0  EquilibriumPositionUnits=deg  SpringStiffness=0  SpringStiffnessUnits=N*m/deg  DampingCoefficient=0  DampingCoefficientUnits=N*m/(deg/s)  TorqueActuationMode=InputTorque  MotionActuationMode=ComputedMotion  SensePosition=off  SenseVelocity=on  SenseAcceleration=off  SenseTorqueForce=off  SenseLowerLimitTorqueForce=off  SenseUpperLimitTorqueForce=off  LowerLimitSpecify=off  LowerLimitBound=-90  LowerLimitBoundUnits=deg  LowerLimitStiffness=1e4  LowerLimitStiffnessUnits=N*m/deg  LowerLimitDamping=10  LowerLimitDampingUnits=N*m/(deg/s)  LowerLimitTransitionRegionWidth=0.1  LowerLimitTransitionRegionWidthUnits=deg  UpperLimitSpecify=off  UpperLimitBound=90  UpperLimitBoundUnits=deg  UpperLimitStiffness=1e4  UpperLimitStiffnessUnits=N*m/deg  UpperLimitDamping=10  UpperLimitDampingUnits=N*m/(deg/s)  UpperLimitTransitionRegionWidth=0.1  UpperLimitTransitionRegionWidthUnits=deg  PositionTargetSpecify=off  PositionTargetPriority=High  PositionTargetValue=0  PositionTargetValueUnits=deg  VelocityTargetSpecify=on  VelocityTargetPriority=High  VelocityTargetValue=0  VelocityTargetValueUnits=rad/s
  Outrunner Motor : sm_lib/Body Elements/Cylindrical Solid  GraphicAmbientColor=[0.15 0.15 0.15 1.0]  BasedOnType=Mass  CenterOfMass=[0 0 0]  CenterOfMassUnits=m  GraphicDiffuseColor=[0.2 0.6 0.0]  CylinderLength=0.05  CylinderLengthUnits=m  CylinderRadius=0.02  CylinderRadiusUnits=m  Density=1000  DensityUnits=kg/(m^3)  DoExposeReferenceFrame=on  GraphicEmissiveColor=[0.0 0.0 0.0 1.0]  ExportEntireGeometry=off  SerializedFrames=<Frames/>  MarkerShape=Sphere  MarkerSize=10  GraphicType=FromGeometry  InertiaType=CalculateFromGeometry  Mass=motorMass  MassUnits=kg  MomentsOfInertia=[1 1 1]  MomentsOfInertiaUnits=kg*m^2  GraphicOpacity=1.0  ProductsOfInertia=[0 0 0]  ProductsOfInertiaUnits=kg*m^2  GraphicShininess=75  GraphicSpecularColor=[0.5 0.5 0.5 1.0]  GraphicVisPropType=SimpleVisualProperties
  PS-Simulink Converter3 : nesl_utility/PS-Simulink Converter  PhysicalDomain=network_engine_domain  SubClassName=ps_output  LeftPortType=input  RightPortType=output  PseudoPeriodic=off  Frequencies=[]  VectorFormat=1-D array  Unit=1  AffineConversion=off
  Product1 : Product
  Product2 : Product
  Product3 : Product
  Product6 : Product  Inputs=3
  Propeller : sm_lib/Body Elements/Brick Solid  GraphicAmbientColor=[0.15 0.15 0.15 1.0]  BasedOnType=Mass  BrickDimensions=[0.34 0.03 0.01]  BrickDimensionsUnits=m  CenterOfMass=[0 0 0]  CenterOfMassUnits=m  GraphicDiffuseColor=[0.9 0 0.0]  Density=1000  DensityUnits=kg/(m^3)  DoExposeReferenceFrame=on  GraphicEmissiveColor=[0.0 0.0 0.0 1.0]  ExportEntireGeometry=off  SerializedFrames=<Frames/>  MarkerShape=Sphere  MarkerSize=10  GraphicType=FromGeometry  InertiaType=CalculateFromGeometry  Mass=propellerMass  MassUnits=kg  MomentsOfInertia=[1 1 1]  MomentsOfInertiaUnits=kg*m^2  GraphicOpacity=1.0  ProductsOfInertia=[0 0 0]  ProductsOfInertiaUnits=kg*m^2  GraphicShininess=75  GraphicSpecularColor=[0.5 0.5 0.5 1.0]  GraphicVisPropType=SimpleVisualProperties
  Rigid Transform1 : sm_lib/Frames and Transforms/Rigid Transform  TranslationMethod=Cartesian  TranslationStandardOffset=0  TranslationStandardOffsetUnits=m  TranslationStandardAxis=+Z  TranslationCartesianOffset=[0 0 0.03]  TranslationCartesianOffsetUnits=m  TranslationROffset=0  TranslationROffsetUnits=m  TranslationZOffset=0  TranslationZOffsetUnits=m  TranslationThetaOffset=0  TranslationThetaOffsetUnits=deg  RotationMethod=StandardAxis  RotationAngleUnits=deg  RotationStandardAxis=+Z  RotationAngle=0.0  RotationArbitraryAxis=[0 0 1]  FollAlignAxisA=+X  BaseAlignAxisA=+Y  FollAlignAxisB=+Y  BaseAlignAxisB=+Z  RotationSequenceAxes=FollowerAxes  RotationSequence=XYX  RotationSequenceAngles=[0 0 0]  RotationSequenceAnglesUnits=deg  RotationMatrix=[1 0 0; 0 1 0; 0 0 1]  Quaternion=[1 0 0 0]
  Simulink-PS Converter1 : nesl_utility/Simulink-PS Converter  PhysicalDomain=network_engine_domain  SubClassName=ps_input  LeftPortType=input  RightPortType=output  PseudoPeriodic=off  Frequencies=[]  NoiseDistribution=none  NoiseParameters=[]  Unit=1  AffineConversion=off  FilteringAndDerivatives=zero  SimscapeFilterOrder=1  InputFilterTimeConstant=0.001  UdotUserProvided=1
  Simulink-PS Converter2 : nesl_utility/Simulink-PS Converter  PhysicalDomain=network_engine_domain  SubClassName=ps_input  LeftPortType=input  RightPortType=output  PseudoPeriodic=off  Frequencies=[]  NoiseDistribution=none  NoiseParameters=[]  Unit=1  AffineConversion=off  FilteringAndDerivatives=zero  SimscapeFilterOrder=1  InputFilterTimeConstant=0.001  UdotUserProvided=1
  Sum : Sum  Inputs=|+-
  Sum2 : Sum  Inputs=|+-
  drag_konstant : Gain  Gain=KDrag
  motor_konstant : Constant  Value=Km
  rad/s to RPM : Gain  Gain=60/2/pi
  trust_konstant : Gain  Gain=Ktrust
  w_squared : Product
  pos : PMIOPort  Side=Left
  RPM : Outport  VectorParamsAs1DForOutWhenUnconnected=off
  trust : Outport  Port=2  VectorParamsAs1DForOutWhenUnconnected=off
  omega : Outport  Port=3  VectorParamsAs1DForOutWhenUnconnected=off
  wires:
  Product6/1 -> drag_konstant/1
  PS-Simulink Converter3/1 -> Product6/1, Product6/2, Product6/3, w_squared/1, w_squared/2, Product1/1, rad/s to RPM/1, omega/1
  w_squared/1 -> trust_konstant/1
  trust_konstant/1 -> Simulink-PS Converter1/1, trust/1
  CV_CCV/1 -> Product3/1
  Product3/1 -> Sum/1
  volt/1 -> Product3/2
  drag_konstant/1 -> Sum2/2
  Sum2/1 -> Simulink-PS Converter2/1
  Sum/1 -> Ankrmodstand/1
  Ankrmodstand/1 -> Dead Zone/1  "motor current"
  Product2/1 -> Sum2/1  "motor torque"
  Product1/1 -> Sum/2
  motor_konstant/1 -> Product1/2, Product2/2
  rad/s to RPM/1 -> RPM/1
  Dead Zone/1 -> Product2/1
  connections:
  Rigid Transform1/RConn1 -- Propeller/RConn1 -- External Force and Torque/RConn1
  pos/RConn1 -- Outrunner Motor/RConn1 -- Motor axle/LConn1
  Simulink-PS Converter2/RConn1 -- Motor axle/LConn2
  Motor axle/RConn1 -- Rigid Transform1/LConn1
  Motor axle/RConn2 -- PS-Simulink Converter3/LConn1
  Simulink-PS Converter1/RConn1 -- External Force and Torque/LConn1

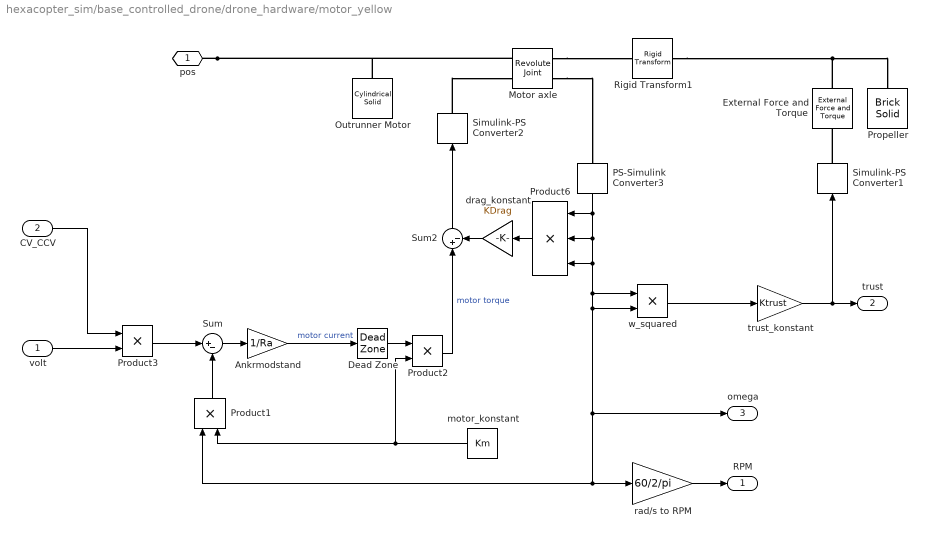
== system hexacopter_sim/base_controlled_drone/drone_hardware/motor_yellow ==
  volt : Inport
  CV_CCV : Inport  Port=2
  Ankrmodstand : Gain  Gain=1/Ra
  Dead Zone : DeadZone  LowerValue=-deadCurrent  UpperValue=deadCurrent
  External Force and Torque : sm_lib/Forces and Torques/External Force and Torque  ForceResolutionFrame=AttachedFrame  EnableForceX=off  EnableForceY=off  EnableForceZ=on  EnableForce=off  TorqueResolutionFrame=AttachedFrame  EnableTorqueX=off  EnableTorqueY=off  EnableTorqueZ=off  EnableTorque=off
  Motor axle : sm_lib/Joints/Revolute Joint  JointMode=Normal  SenseConstraintForce=off  SenseConstraintForceX=off  SenseConstraintForceY=off  SenseConstraintForceZ=off  SenseConstraintTorque=off  SenseConstraintTorqueX=off  SenseConstraintTorqueY=off  SenseConstraintTorqueZ=off  SenseTotalForce=off  SenseTotalForceX=off  SenseTotalForceY=off  SenseTotalForceZ=off  SenseTotalTorque=off  SenseTotalTorqueX=off  SenseTotalTorqueY=off  SenseTotalTorqueZ=off  CompositeWrenchDir=FollowerOnBase  CompositeWrenchFrame=BaseFrame  EquilibriumPosition=0  EquilibriumPositionUnits=deg  SpringStiffness=0  SpringStiffnessUnits=N*m/deg  DampingCoefficient=0  DampingCoefficientUnits=N*m/(deg/s)  TorqueActuationMode=InputTorque  MotionActuationMode=ComputedMotion  SensePosition=off  SenseVelocity=on  SenseAcceleration=off  SenseTorqueForce=off  SenseLowerLimitTorqueForce=off  SenseUpperLimitTorqueForce=off  LowerLimitSpecify=off  LowerLimitBound=-90  LowerLimitBoundUnits=deg  LowerLimitStiffness=1e4  LowerLimitStiffnessUnits=N*m/deg  LowerLimitDamping=10  LowerLimitDampingUnits=N*m/(deg/s)  LowerLimitTransitionRegionWidth=0.1  LowerLimitTransitionRegionWidthUnits=deg  UpperLimitSpecify=off  UpperLimitBound=90  UpperLimitBoundUnits=deg  UpperLimitStiffness=1e4  UpperLimitStiffnessUnits=N*m/deg  UpperLimitDamping=10  UpperLimitDampingUnits=N*m/(deg/s)  UpperLimitTransitionRegionWidth=0.1  UpperLimitTransitionRegionWidthUnits=deg  PositionTargetSpecify=off  PositionTargetPriority=High  PositionTargetValue=0  PositionTargetValueUnits=deg  VelocityTargetSpecify=on  VelocityTargetPriority=High  VelocityTargetValue=0  VelocityTargetValueUnits=rad/s
  Outrunner Motor : sm_lib/Body Elements/Cylindrical Solid  GraphicAmbientColor=[0.15 0.15 0.15 1.0]  BasedOnType=Mass  CenterOfMass=[0 0 0]  CenterOfMassUnits=m  GraphicDiffuseColor=[0.2 0.6 0.0]  CylinderLength=0.05  CylinderLengthUnits=m  CylinderRadius=0.02  CylinderRadiusUnits=m  Density=1000  DensityUnits=kg/(m^3)  DoExposeReferenceFrame=on  GraphicEmissiveColor=[0.0 0.0 0.0 1.0]  ExportEntireGeometry=off  SerializedFrames=<Frames/>  MarkerShape=Sphere  MarkerSize=10  GraphicType=FromGeometry  InertiaType=CalculateFromGeometry  Mass=motorMass  MassUnits=kg  MomentsOfInertia=[1 1 1]  MomentsOfInertiaUnits=kg*m^2  GraphicOpacity=1.0  ProductsOfInertia=[0 0 0]  ProductsOfInertiaUnits=kg*m^2  GraphicShininess=75  GraphicSpecularColor=[0.5 0.5 0.5 1.0]  GraphicVisPropType=SimpleVisualProperties
  PS-Simulink Converter3 : nesl_utility/PS-Simulink Converter  PhysicalDomain=network_engine_domain  SubClassName=ps_output  LeftPortType=input  RightPortType=output  PseudoPeriodic=off  Frequencies=[]  VectorFormat=1-D array  Unit=1  AffineConversion=off
  Product1 : Product
  Product2 : Product
  Product3 : Product
  Product6 : Product  Inputs=3
  Propeller : sm_lib/Body Elements/Brick Solid  GraphicAmbientColor=[0.15 0.15 0.15 1.0]  BasedOnType=Mass  BrickDimensions=[0.34 0.03 0.01]  BrickDimensionsUnits=m  CenterOfMass=[0 0 0]  CenterOfMassUnits=m  GraphicDiffuseColor=[0.8 0.8 0.0]  Density=1000  DensityUnits=kg/(m^3)  DoExposeReferenceFrame=on  GraphicEmissiveColor=[0.0 0.0 0.0 1.0]  ExportEntireGeometry=off  SerializedFrames=<Frames/>  MarkerShape=Sphere  MarkerSize=10  GraphicType=FromGeometry  InertiaType=CalculateFromGeometry  Mass=propellerMass  MassUnits=kg  MomentsOfInertia=[1 1 1]  MomentsOfInertiaUnits=kg*m^2  GraphicOpacity=1.0  ProductsOfInertia=[0 0 0]  ProductsOfInertiaUnits=kg*m^2  GraphicShininess=75  GraphicSpecularColor=[0.5 0.5 0.5 1.0]  GraphicVisPropType=SimpleVisualProperties
  Rigid Transform1 : sm_lib/Frames and Transforms/Rigid Transform  TranslationMethod=Cartesian  TranslationStandardOffset=0  TranslationStandardOffsetUnits=m  TranslationStandardAxis=+Z  TranslationCartesianOffset=[0 0 0.03]  TranslationCartesianOffsetUnits=m  TranslationROffset=0  TranslationROffsetUnits=m  TranslationZOffset=0  TranslationZOffsetUnits=m  TranslationThetaOffset=0  TranslationThetaOffsetUnits=deg  RotationMethod=StandardAxis  RotationAngleUnits=deg  RotationStandardAxis=+Z  RotationAngle=0.0  RotationArbitraryAxis=[0 0 1]  FollAlignAxisA=+X  BaseAlignAxisA=+Y  FollAlignAxisB=+Y  BaseAlignAxisB=+Z  RotationSequenceAxes=FollowerAxes  RotationSequence=XYX  RotationSequenceAngles=[0 0 0]  RotationSequenceAnglesUnits=deg  RotationMatrix=[1 0 0; 0 1 0; 0 0 1]  Quaternion=[1 0 0 0]
  Simulink-PS Converter1 : nesl_utility/Simulink-PS Converter  PhysicalDomain=network_engine_domain  SubClassName=ps_input  LeftPortType=input  RightPortType=output  PseudoPeriodic=off  Frequencies=[]  NoiseDistribution=none  NoiseParameters=[]  Unit=1  AffineConversion=off  FilteringAndDerivatives=zero  SimscapeFilterOrder=1  InputFilterTimeConstant=0.001  UdotUserProvided=1
  Simulink-PS Converter2 : nesl_utility/Simulink-PS Converter  PhysicalDomain=network_engine_domain  SubClassName=ps_input  LeftPortType=input  RightPortType=output  PseudoPeriodic=off  Frequencies=[]  NoiseDistribution=none  NoiseParameters=[]  Unit=1  AffineConversion=off  FilteringAndDerivatives=zero  SimscapeFilterOrder=1  InputFilterTimeConstant=0.001  UdotUserProvided=1
  Sum : Sum  Inputs=|+-
  Sum2 : Sum  Inputs=|+-
  drag_konstant : Gain  Gain=KDrag
  motor_konstant : Constant  Value=Km
  rad/s to RPM : Gain  Gain=60/2/pi
  trust_konstant : Gain  Gain=Ktrust
  w_squared : Product
  pos : PMIOPort  Side=Left
  RPM : Outport  VectorParamsAs1DForOutWhenUnconnected=off
  trust : Outport  Port=2  VectorParamsAs1DForOutWhenUnconnected=off
  omega : Outport  Port=3  VectorParamsAs1DForOutWhenUnconnected=off
  wires:
  Product6/1 -> drag_konstant/1
  PS-Simulink Converter3/1 -> Product6/1, Product6/2, Product6/3, w_squared/1, w_squared/2, Product1/1, rad/s to RPM/1, omega/1
  w_squared/1 -> trust_konstant/1
  trust_konstant/1 -> Simulink-PS Converter1/1, trust/1
  CV_CCV/1 -> Product3/1
  Product3/1 -> Sum/1
  volt/1 -> Product3/2
  drag_konstant/1 -> Sum2/2
  Sum2/1 -> Simulink-PS Converter2/1
  Sum/1 -> Ankrmodstand/1
  Ankrmodstand/1 -> Dead Zone/1  "motor current"
  Product2/1 -> Sum2/1  "motor torque"
  Product1/1 -> Sum/2
  motor_konstant/1 -> Product1/2, Product2/2
  rad/s to RPM/1 -> RPM/1
  Dead Zone/1 -> Product2/1
  connections:
  Rigid Transform1/RConn1 -- Propeller/RConn1 -- External Force and Torque/RConn1
  pos/RConn1 -- Outrunner Motor/RConn1 -- Motor axle/LConn1
  Simulink-PS Converter2/RConn1 -- Motor axle/LConn2
  Motor axle/RConn1 -- Rigid Transform1/LConn1
  Motor axle/RConn2 -- PS-Simulink Converter3/LConn1
  Simulink-PS Converter1/RConn1 -- External Force and Torque/LConn1

== system hexacopter_sim/base_controlled_drone/platform/Dæmpet understel ==
  note: Dæmpet understel
  Heingt_rate : Inport
  Height : Inport  Port=2
  Gain : Gain  Gain=-1000
  Gain1 : Gain  Gain=0.2
  Saturation : Saturate  UpperLimit=0
  Saturation1 : Saturate  UpperLimit=0.2  LowerLimit=-0.2
  Sum : Sum  Inputs=+|+-
  dist_above_gnd : Constant  Value=0.0
  Ground_N : Outport  VectorParamsAs1DForOutWhenUnconnected=off
  wires:
  Height/1 -> Sum/2
  Sum/1 -> Saturation/1
  Gain1/1 -> Sum/1
  Saturation1/1 -> Gain1/1
  Gain/1 -> Ground_N/1
  Saturation/1 -> Gain/1
  Heingt_rate/1 -> Saturation1/1
  dist_above_gnd/1 -> Sum/3
